simulink model "single_pend_linear"  (R2015a)
settings: Solver=ode45  StartTime=0.0  StopTime=5  RelTol=1e-3
PreLoadFcn:
  | single_pend
InitFcn:
  | single_pend
StartFcn:
  | single_pend
values from neighbouring files (symbols this model uses):
  a = 0.1    [double_pend_feedback.m]    (also in fuzzy_logic.m; single_pend.m)
  A_ = [0 1 0 0; -k/mass -damper/mass (sqrt(ep*2*a*k))/ep*a*mass 0; 0 0 0 1; 0 0 0 -R/L]    [double_pend_feedback.m]    (also in fuzzy_logic.m; single_pend.m)
  b = 0.1    [single_pend.m]
  B_ = [0; 1/mass; 0;0]    [double_pend_feedback.m]    (also in fuzzy_logic.m; single_pend.m)
  damper = 200    [double_pend_feedback.m]    (also in fuzzy_logic.m; single_pend.m)
  ep = 1    [double_pend_feedback.m]    (also in fuzzy_logic.m; single_pend.m)
  g = 9.81    [single_pend.m]
  k = 1    [double_pend_feedback.m]    (also in fuzzy_logic.m; single_pend.m)
  KA = K_non_rep    [single_pend.m]
  l = 0.3    [single_pend.m]
  L = 0.0001    [double_pend_feedback.m]    (also in fuzzy_logic.m; single_pend.m)
  m = 0.2    [single_pend.m]
  M = 1    [single_pend.m]
  mass = 0.5    [double_pend_feedback.m]    (also in fuzzy_logic.m; single_pend.m)
  R = 100    [double_pend_feedback.m]    (also in fuzzy_logic.m; single_pend.m)
libraries: simulink x1
settings Model: Creator=Nabeel  LastModifiedBy=Nabeel

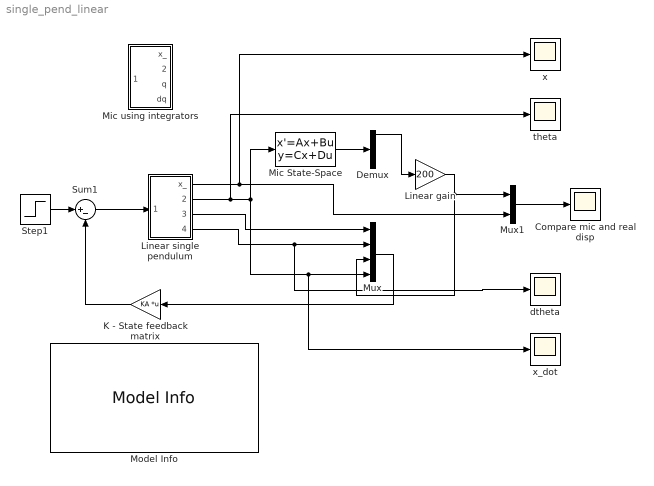
== system single_pend_linear ==
  Compare mic and real disp : Scope
      settings: ShowLegends=on  YMin=-0.01  YMax=0.13
  Demux : Demux
  K - State feedback matrix : Gain  Gain=KA  Multiplication=Matrix(K*u)
  Linear gain : Gain  Gain=200
  Linear single pendulum : Subsystem
  Mic State-Space : StateSpace  A=A_  B=B_  C=eye(4)  D=[0;0;0;0]  X0=0
  Mic using integrators : Subsystem
  Model Info : simulink/Model-Wide Utilities/Model Info  Frame=on  DisplayStringWithTags=|  HorizontalTextAlignment=Center  LeftAlignmentValue=0.5  SourceBlockDiagram=single_pend_linear  TagMaxNumber=20
      | State feedback matrix info:
      | Replace the feedback block to test others
      | Gain block
      | KA- pole placement (repeated)
      | KB - pole placement (non-repeated)
      | K1 - LQR 1 
      | K2 - LQR 2
      | K3 - LQR 3
      | K4 - LQR 4
  Mux : Mux
  Mux1 : Mux  Inputs=2
  Step1 : Step  SampleTime=0
  Sum1 : Sum  Inputs=|+-
  dtheta : Scope
      settings: SaveName=dtheta
  theta : Scope
      settings: ShowLegends=on  SaveName=theta
  x : Scope
      settings: ShowLegends=on  SaveName=x
  x_dot : Scope
      settings: ShowLegends=on  YMin=-0.1044  YMax=-0.10395  SaveName=xdot
  wires:
  Mux/1 -> K - State feedback matrix/1
  Linear single pendulum/3(theta) -> Mux/1
  Demux/1 -> Linear gain/1
  Linear single pendulum/4(dtheta) -> Mux/2, dtheta/1
  Step1/1 -> Sum1/1
  K - State feedback matrix/1 -> Sum1/2
  Sum1/1 -> Linear single pendulum/1(In1)
  Mic State-Space/1 -> Demux/1
  Linear single pendulum/1(x_) -> x/1, Mux1/2
  Linear single pendulum/2(x_dot) -> theta/1, x_dot/1, Mux/4, Mic State-Space/1
  Mux1/1 -> Compare mic and real disp/1
  Linear gain/1 -> Mux1/1, Mux/3

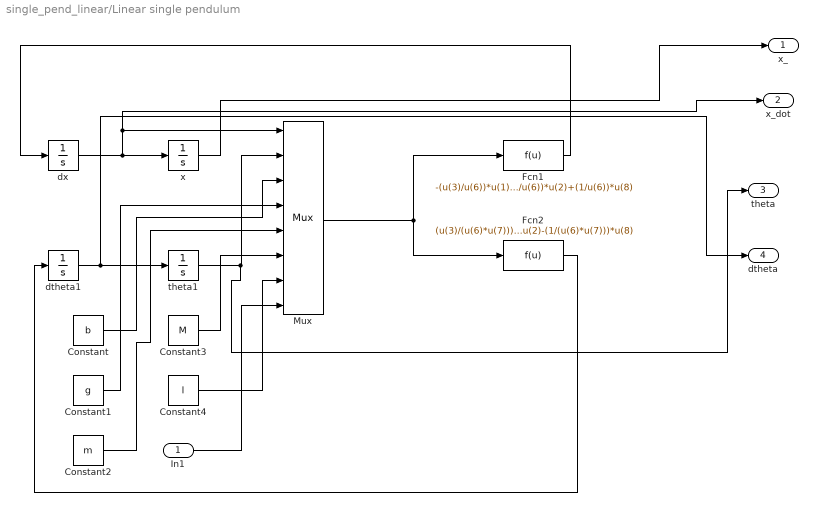
== system single_pend_linear/Linear single pendulum ==
  In1 : Inport
  Constant : Constant  Value=b
  Constant1 : Constant  Value=g
  Constant2 : Constant  Value=m
  Constant3 : Constant  Value=M
  Constant4 : Constant  Value=l
  Fcn1 : Fcn  Expr=-(u(3)/u(6))*u(1)-((u(4)*u(5))/u(6))*u(2)+(1/u(6))*u(8)
  Fcn2 : Fcn  Expr=(u(3)/(u(6)*u(7)))*u(1)+((u(4)*(u(5)+u(6)))/(u(6)*u(7)))*u(2)-(1/(u(6)*u(7)))*u(8)
  Mux : Mux  Inputs=8
  dtheta1 : Integrator
  dx : Integrator
  theta1 : Integrator  UpperSaturationLimit=3.14  LowerSaturationLimit=-3.14
  x : Integrator
  x_ : Outport
  x_dot : Outport  Port=2
  theta : Outport  Port=3
  dtheta : Outport  Port=4
  wires:
  dtheta1/1 -> dtheta/1, theta1/1
  Constant3/1 -> Mux/6
  dx/1 -> x_dot/1, Mux/1, x/1
  Fcn1/1 -> dx/1
  Constant1/1 -> Mux/4
  Constant4/1 -> Mux/7
  In1/1 -> Mux/8
  Constant/1 -> Mux/3
  x/1 -> x_/1
  Mux/1 -> Fcn1/1, Fcn2/1
  Constant2/1 -> Mux/5
  theta1/1 -> theta/1, Mux/2
  Fcn2/1 -> dtheta1/1

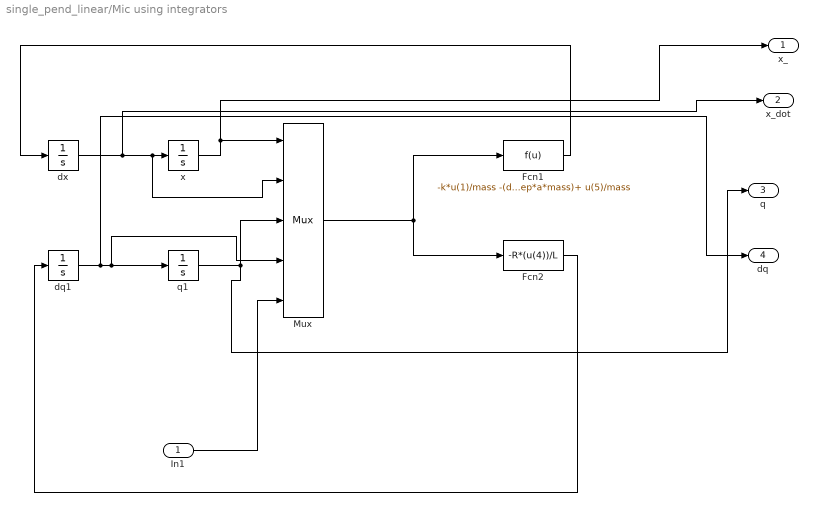
== system single_pend_linear/Mic using integrators ==
  In1 : Inport
  Fcn1 : Fcn  Expr=-k*u(1)/mass -(damper*u(2))/mass +(u(3))*((sqrt(ep*2*a*k))/ep*a*mass)+ u(5)/mass
  Fcn2 : Fcn  Expr=-R*(u(4))/L
  Mux : Mux  Inputs=5
  dq1 : Integrator
  dx : Integrator
  q1 : Integrator  InitialCondition=0.01  UpperSaturationLimit=3.14  LowerSaturationLimit=-3.14
  x : Integrator
  x_ : Outport
  x_dot : Outport  Port=2
  q : Outport  Port=3
  dq : Outport  Port=4
  wires:
  Fcn1/1 -> dx/1
  x/1 -> Mux/1, x_/1
  Mux/1 -> Fcn1/1, Fcn2/1
  q1/1 -> q/1, Mux/3
  Fcn2/1 -> dq1/1
  dq1/1 -> Mux/4, q1/1, dq/1
  dx/1 -> x_dot/1, Mux/2, x/1
  In1/1 -> Mux/5
